simulink model "shared_gas_burner"  (R2021a)
settings: Solver=FixedStepAuto  StartTime=0.0  StopTime=timeFinal  FixedStep=timeStepMax  MaxStep=timeStepMax  RelTol=1e-3
model workspace (MAT data in the model file):
  initX1 = 0
  initX2 = 50
values from neighbouring files (symbols this model uses):
  a_init = x0_0    [run_SharedGasBurner.m]
  b_init = x1_0    [run_SharedGasBurner.m]
settings Model: OrderedModelArguments=off  Creator=calros  LastModifiedBy=amit
settings SolverCC: AlgebraicLoopSolver=TrustRegion
settings DataIOCC: SaveFormat=Structure
settings DebuggingCC: SFMachineParentedDataDiag=warning  UnderSpecifiedDimensionMsg=error
settings SFSimCC: CustomCodeUndefinedFunction=UseInterfaceOnly

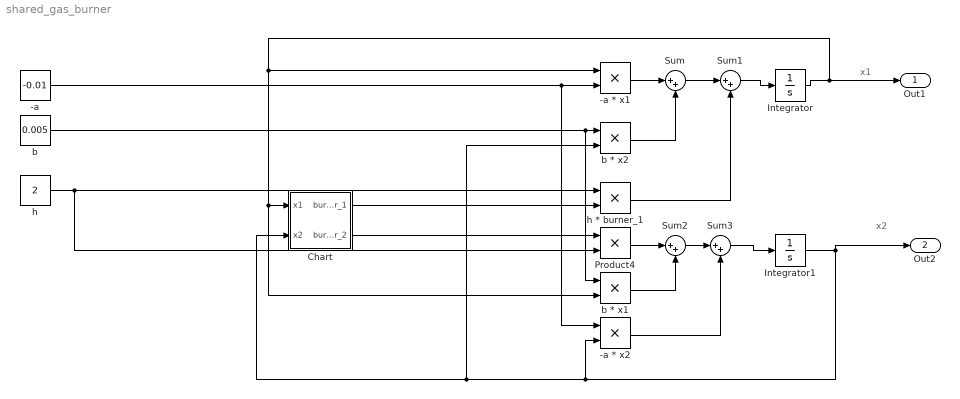
== system shared_gas_burner ==
  note: x1
  note: x2
  -a : Constant  Value=-0.01
  -a * x1 : Product
  -a * x2 : Product
  Chart : Stateflow chart  TreatAsAtomicUnit=on
  Integrator : Integrator  InitialCondition=a_init
  Integrator1 : Integrator  InitialCondition=b_init
  Product4 : Product
  Sum{,1..3} (4 alike) : Sum  Inputs=|++
  b : Constant  Value=0.005
  b * x1 : Product
  b * x2 : Product
  h : Constant  Value=2
  h * burner_1 : Product
  Out1 : Outport  VectorParamsAs1DForOutWhenUnconnected=off
  Out2 : Outport  Port=2  VectorParamsAs1DForOutWhenUnconnected=off
  wires:
  Integrator/1 -> Out1/1, -a * x1/1, b * x1/2, Chart/1(x1)
  -a/1 -> -a * x1/2, -a * x2/1
  Integrator1/1 -> Out2/1, -a * x2/2, b * x2/2, Chart/2(x2)
  b/1 -> b * x1/1, b * x2/1
  h/1 -> Product4/2, h * burner_1/1
  Chart/1(burner_1) -> h * burner_1/2
  -a * x1/1 -> Sum/1
  b * x2/1 -> Sum/2
  h * burner_1/1 -> Sum1/2
  Sum1/1 -> Integrator/1
  Sum/1 -> Sum1/1
  Chart/2(burner_2) -> Product4/1
  Product4/1 -> Sum2/1
  Sum3/1 -> Integrator1/1
  Sum2/1 -> Sum3/1
  -a * x2/1 -> Sum3/2
  b * x1/1 -> Sum2/2

== stateflow chart shared_gas_burner/Chart ==
  state l1
    burner_1 = 1;
    burner_2 = 0;
  state l0
    burner_1 = 0;
    burner_2 = 0;
  state l2
    burner_1 = 0;
    burner_2 = 1;
  l1 -> l2 [order 1] : [(x1 <= 80 && x2 >= 100)]
  (default) -> l1
  l1 -> l0 [order 2] : [x1>=100]
  l0 -> l2 [order 2] : [x2 <= 80]
  l2 -> l0 [order 2] : [x2 >= 100]
  l0 -> l1 [order 1] : [x1<=80]
  l2 -> l1 [order 1] : [(x2 >= 20 && x1 <= 0)]
  data: x1 input; x2 input; burner_1 output; burner_2 output
